simulink model "CM620C_MotAg0Meas"  (R2013b)
settings: Solver=FixedStepDiscrete  SolverMode=SingleTasking  StartTime=0.0  StopTime=1  FixedStep=0.0000625  RelTol=1e-3
values from neighbouring files (symbols this model uses):
  ARCHGLBPRM_2PI_ULS_F32 = DataDict.Constant    [CM620C_MotAg0Meas_DataDict.m]
  COEFFTBLELMSIZE_CNT_U08 = DataDict.Constant    [CM620C_MotAg0Meas_DataDict.m]
  COEFFTBLSIZE_CNT_U08 = DataDict.Constant    [CM620C_MotAg0Meas_DataDict.m]
  CORRNTBLAGSTEPSIZE_MATRAD_F32 = DataDict.Constant    [CM620C_MotAg0Meas_DataDict.m]
  CORRNTBLSIDXOFFS_CNT_U16 = DataDict.Constant    [CM620C_MotAg0Meas_DataDict.m]
  CORRNTBLSIZE_CNT_U16 = DataDict.Constant    [CM620C_MotAg0Meas_DataDict.m]
  CORRNTBLSIZEMASK_CNT_U08 = DataDict.Constant    [CM620C_MotAg0Meas_DataDict.m]
  MOTAG0ERRTHD_MOTREV_U0P16 = DataDict.Constant    [CM620C_MotAg0Meas_DataDict.m]
  MotAg0PrtclFlt = DataDict.NTC    [CM620C_MotAg0Meas_DataDict.m]
  MOTAG0PRTCLFLTFAILSTEP_CNT_U16 = DataDict.Constant    [CM620C_MotAg0Meas_DataDict.m]
  MOTAG0PRTCLFLTPASSSTEP_CNT_U16 = DataDict.Constant    [CM620C_MotAg0Meas_DataDict.m]
  MOTAGCPTLIMFLTMASK_CNT_U32 = DataDict.Constant    [CM620C_MotAg0Meas_DataDict.m]
  MOTAGDELTAPERCORRNPT_CNT_U16 = DataDict.Constant    [CM620C_MotAg0Meas_DataDict.m]
  MOTAGFLTMASK_CNT_U32 = DataDict.Constant    [CM620C_MotAg0Meas_DataDict.m]
  MOTAGIDXMASK_CNT_U16 = DataDict.Constant    [CM620C_MotAg0Meas_DataDict.m]
  MOTAGLIMMASK_CNT_S32 = DataDict.Constant    [CM620C_MotAg0Meas_DataDict.m]
  MOTAGMGNLIMFLTMASK_CNT_U32 = DataDict.Constant    [CM620C_MotAg0Meas_DataDict.m]
  MOTAGMINWAITPERD_CNT_U32 = DataDict.Constant    [CM620C_MotAg0Meas_DataDict.m]
  MOTAGOFFS_CNT_S32 = DataDict.Constant    [CM620C_MotAg0Meas_DataDict.m]
  MOTAGOVFFLTMASK_CNT_U32 = DataDict.Constant    [CM620C_MotAg0Meas_DataDict.m]
  MOTAGSPITRSMMASK_CNT_U32 = DataDict.Constant    [CM620C_MotAg0Meas_DataDict.m]
  MOTAGVLTGFLTMASK_CNT_U32 = DataDict.Constant    [CM620C_MotAg0Meas_DataDict.m]
  NOMOTAGFLTMASK_CNT_U32 = DataDict.Constant    [CM620C_MotAg0Meas_DataDict.m]
  READBUFADR_CNT_U32 = DataDict.Constant    [CM620C_MotAg0Meas_DataDict.m]
  READBUFIDX_CNT_U08 = DataDict.Constant    [CM620C_MotAg0Meas_DataDict.m]
  SNSRAGMASK_CNT_U32 = DataDict.Constant    [CM620C_MotAg0Meas_DataDict.m]
  SNSRCNTMASK_CNT_U32 = DataDict.Constant    [CM620C_MotAg0Meas_DataDict.m]
  SPIAGCNTREGIDX_CNT_U08 = DataDict.Constant    [CM620C_MotAg0Meas_DataDict.m]
  SPIAGREGIDX_CNT_U08 = DataDict.Constant    [CM620C_MotAg0Meas_DataDict.m]
  SPISTATREGIDX_CNT_U08 = DataDict.Constant    [CM620C_MotAg0Meas_DataDict.m]
  SPITURNCNTRREGIDX_CNT_U08 = DataDict.Constant    [CM620C_MotAg0Meas_DataDict.m]
  STRTPTRINITVAL_CNT_U32 = DataDict.Constant    [CM620C_MotAg0Meas_DataDict.m]
  STRTPTRPERVAL_CNT_U32 = DataDict.Constant    [CM620C_MotAg0Meas_DataDict.m]
  TURNCNTRHALFOFFS_CNT_S16 = DataDict.Constant    [CM620C_MotAg0Meas_DataDict.m]
  TURNCNTROFFS_CNT_S16 = DataDict.Constant    [CM620C_MotAg0Meas_DataDict.m]
  TURNCNTRREGMASK_CNT_U32 = DataDict.Constant    [CM620C_MotAg0Meas_DataDict.m]
  VLDMOTAGFLTMASK_CNT_U32 = DataDict.Constant    [CM620C_MotAg0Meas_DataDict.m]
undefined symbols (not defined in the file or in its folder): NtcSts1, sigbuilder_block
libraries: simulink x41, FloatToFixd x1, NxtrMax x1
(part 4 of 7)

== system CM620C_MotAg0Meas/MotAg0Meas/MotAg0MeasPer2/MotAg0Calcn/MotAg0Processing/Offset Compensation /Rt Offs Calcn ==
  MotAg3Mecl : Inport  RequirementInfo={} %GIDa_68f0f226_5b53_4cfc_a377_050a14e64919
  MotAg0SpiMecl : Inport  RequirementInfo={} %GIDa_5deca769_324c_4965_b2f5_c5a430060931  Port=2
  Action Port : ActionPort  ActionType=else
  CopyRight2 : Subsystem  Description=|  mask(Copyright Information){none=on}
      | Copyright info block.                                               
      |                                                                     
      | Place copyright information at the top of every subsystem in design.
      mask prompts: none "No parameters"
      mask help: Place copyright information at the top of every subsystem in design.
      mask Display:
      | NxtrConf = 'Nexteer Confidential';
      | 
      | sys = bdroot; %handle for the current model ("system")
      | first = get_param(sys,'Created');
      | first = first(end-3:end);  %year is last four digits
      | 
      | last = get_param(sys,'LastModifiedDate');
      | if isempty(last)
      |     last = datestr(now,'yyyy');
      | else
      |     last = last(end-3:end);
      | end
      | 
      | if strcmp(first,last)
      |     fprintf('%s -- Copyright %s Nexteer',NxtrConf,first)
      | else
      |     fprintf('%s -- %s%s- %s Nexteer',NxtrConf,char(169),first,last)
      | end
  Data Store Read1 : DataStoreRead  DataStoreName=MotAg0PrevOffs
  Data Type Conversion : DataTypeConversion  OutDataTypeStr=int32
  Data Type Conversion1 : DataTypeConversion  OutDataTypeStr=int32
  Subtract : Sum  Inputs=+-
  MotAg0Offs : Outport
  MotAg0RtOffs : Outport  Port=2
  wires:
  MotAg3Mecl/1 -> Data Type Conversion/1
  Subtract/1 -> MotAg0RtOffs/1
  Data Type Conversion1/1 -> Subtract/2
  Data Type Conversion/1 -> Subtract/1
  MotAg0SpiMecl/1 -> Data Type Conversion1/1
  Data Store Read1/1 -> MotAg0Offs/1

== system CM620C_MotAg0Meas/MotAg0Meas/MotAg0MeasPer2/MotAg0Calcn/MotAg0Processing/SPI  Motor Angle Calcn/CopyRight1 ==

== system CM620C_MotAg0Meas/MotAg0Meas/MotAg0MeasPer2/MotAg0Calcn/MotAg0Processing/SPI  Motor Angle Calcn/Polarity Correction ==
  MotAg0RawSpiMecl : Inport
  MotAgMecl0Polarity : Inport  Port=2
  CopyRight1 : Subsystem  Description=|  mask(Copyright Information){none=on}
      | Copyright info block.                                               
      |                                                                     
      | Place copyright information at the top of every subsystem in design.
      mask prompts: none "No parameters"
      mask help: Place copyright information at the top of every subsystem in design.
      mask Display:
      | NxtrConf = 'Nexteer Confidential';
      | 
      | sys = bdroot; %handle for the current model ("system")
      | first = get_param(sys,'Created');
      | first = first(end-3:end);  %year is last four digits
      | 
      | last = get_param(sys,'LastModifiedDate');
      | if isempty(last)
      |     last = datestr(now,'yyyy');
      | else
      |     last = last(end-3:end);
      | end
      | 
      | if strcmp(first,last)
      |     fprintf('%s -- Copyright %s Nexteer',NxtrConf,first)
      | else
      |     fprintf('%s -- %s%s- %s Nexteer',NxtrConf,char(169),first,last)
      | end
  Data Store Write : DataStoreWrite  DataStoreName=dMotAg0MeasMotAg0SpiMecl
  If : If  IfExpression=u1 < 0
  Merge : Merge
  Negative Polarity : Subsystem  TreatAsAtomicUnit=on
  Positive Polarity : Subsystem  TreatAsAtomicUnit=on
  MotAg0SpiMecl : Outport
  wires:
  MotAgMecl0Polarity/1 -> If/1
  MotAg0RawSpiMecl/1 -> Negative Polarity/1(MotAg0RawSpiMecl), Positive Polarity/1(MotAg0RawSpiMecl)
  If/1 -> Negative Polarity/Action
  If/2 -> Positive Polarity/Action
  Negative Polarity/1(MotAg0SpiPolarityCorrd) -> Merge/1
  Positive Polarity/1(MotAg0SpiPolarityCorrd) -> Merge/2
  Merge/1 -> MotAg0SpiMecl/1, Data Store Write/1

== system CM620C_MotAg0Meas/MotAg0Meas/MotAg0MeasPer2/MotAg0Calcn/MotAg0Processing/SPI IIF Motor Angle/CopyRight2 ==

== system CM620C_MotAg0Meas/MotAg0Meas/MotAg0MeasPer2/MotAg0Calcn/MotAg0Processing/SPI IIF Motor Angle/SpiMotAgCnt ==
  note: Square Pulse per angle step. 14 bit- 16384 steps per full roation
  MotAg0AgCntReg : Inport
  14-bit Count Value : simulink/Logic and Bit Operations/Bitwise Operator  logicop=AND  UseBitMask=off  NumInputPorts=2  BitMask=SNSRVLTGFLTMASK_CNT_U32  BitMaskRealWorld=Stored Integer
  16383 : Constant  Value=SNSRCNTMASK_CNT_U32
  CopyRight2 : Subsystem  Description=|  mask(Copyright Information){none=on}
      | Copyright info block.                                               
      |                                                                     
      | Place copyright information at the top of every subsystem in design.
      mask prompts: none "No parameters"
      mask help: Place copyright information at the top of every subsystem in design.
      mask Display:
      | NxtrConf = 'Nexteer Confidential';
      | 
      | sys = bdroot; %handle for the current model ("system")
      | first = get_param(sys,'Created');
      | first = first(end-3:end);  %year is last four digits
      | 
      | last = get_param(sys,'LastModifiedDate');
      | if isempty(last)
      |     last = datestr(now,'yyyy');
      | else
      |     last = last(end-3:end);
      | end
      | 
      | if strcmp(first,last)
      |     fprintf('%s -- Copyright %s Nexteer',NxtrConf,first)
      | else
      |     fprintf('%s -- %s%s- %s Nexteer',NxtrConf,char(169),first,last)
      | end
  Data Type Conversion : DataTypeConversion  OutDataTypeStr=uint16
  Left Shift 2 Bits - p16 : ArithShift  BitShiftNumber=2  BitShiftDirection=Left
  Scope : Scope  NumInputPorts=2
      settings: YMin=0~0  YMax=17000~70000  SaveName=ScopeData4
  MotAg0SpiCntr : Outport
  wires:
  MotAg0AgCntReg/1 -> 14-bit Count Value/1
  16383/1 -> 14-bit Count Value/2
  14-bit Count Value/1 -> Data Type Conversion/1
  Left Shift 2 Bits - p16/1 -> MotAg0SpiCntr/1, Scope/2
  Data Type Conversion/1 -> Left Shift 2 Bits - p16/1, Scope/1

== system CM620C_MotAg0Meas/MotAg0Meas/MotAg0MeasPer2/MotAg0Calcn/MotAg0Processing/Turns Counter Calcn/CopyRight2 ==

== system CM620C_MotAg0Meas/MotAg0Meas/MotAg0MeasPer2/MotAg0Calcn/MotAg0Processing/Turns Counter Calcn/Negative Number ==
  Action Port : ActionPort  ActionType=then
  512 : Constant  Value=TURNCNTROFFS_CNT_S16
  CopyRight2 : Subsystem  Description=|  mask(Copyright Information){none=on}
      | Copyright info block.                                               
      |                                                                     
      | Place copyright information at the top of every subsystem in design.
      mask prompts: none "No parameters"
      mask help: Place copyright information at the top of every subsystem in design.
      mask Display:
      | NxtrConf = 'Nexteer Confidential';
      | 
      | sys = bdroot; %handle for the current model ("system")
      | first = get_param(sys,'Created');
      | first = first(end-3:end);  %year is last four digits
      | 
      | last = get_param(sys,'LastModifiedDate');
      | if isempty(last)
      |     last = datestr(now,'yyyy');
      | else
      |     last = last(end-3:end);
      | end
      | 
      | if strcmp(first,last)
      |     fprintf('%s -- Copyright %s Nexteer',NxtrConf,first)
      | else
      |     fprintf('%s -- %s%s- %s Nexteer',NxtrConf,char(169),first,last)
      | end
  Out1 : Outport
  wires:
  512/1 -> Out1/1

== system CM620C_MotAg0Meas/MotAg0Meas/MotAg0MeasPer2/MotAg0Calcn/MotAg0Processing/Turns Counter Calcn/Positive Number ==
  Action Port : ActionPort  ActionType=else
  Constant3 : Constant  Value=0  OutDataTypeStr=int16
  CopyRight2 : Subsystem  Description=|  mask(Copyright Information){none=on}
      | Copyright info block.                                               
      |                                                                     
      | Place copyright information at the top of every subsystem in design.
      mask prompts: none "No parameters"
      mask help: Place copyright information at the top of every subsystem in design.
      mask Display:
      | NxtrConf = 'Nexteer Confidential';
      | 
      | sys = bdroot; %handle for the current model ("system")
      | first = get_param(sys,'Created');
      | first = first(end-3:end);  %year is last four digits
      | 
      | last = get_param(sys,'LastModifiedDate');
      | if isempty(last)
      |     last = datestr(now,'yyyy');
      | else
      |     last = last(end-3:end);
      | end
      | 
      | if strcmp(first,last)
      |     fprintf('%s -- Copyright %s Nexteer',NxtrConf,first)
      | else
      |     fprintf('%s -- %s%s- %s Nexteer',NxtrConf,char(169),first,last)
      | end
  Out1 : Outport
  wires:
  Constant3/1 -> Out1/1

== system CM620C_MotAg0Meas/MotAg0Meas/MotAg0MeasPer2/MotAg0Calcn/SpiRx/Data/CopyRight2 ==

== system CM620C_MotAg0Meas/MotAg0Meas/MotAg0MeasPer3/Initial Check/IdleState SendTx/Flt Cntr Ena/CopyRight2 ==

== system CM620C_MotAg0Meas/MotAg0Meas/MotAg0MeasPer3/Initial Check/IdleState SendTx/Flt Cntr Ena/Wrap back to 0 ==
  Action Port : ActionPort  ActionType=then
  Constant : Constant  Value=0  OutDataTypeStr=uint16
  CopyRight2 : Subsystem  Description=|  mask(Copyright Information){none=on}
      | Copyright info block.                                               
      |                                                                     
      | Place copyright information at the top of every subsystem in design.
      mask prompts: none "No parameters"
      mask help: Place copyright information at the top of every subsystem in design.
      mask Display:
      | NxtrConf = 'Nexteer Confidential';
      | 
      | sys = bdroot; %handle for the current model ("system")
      | first = get_param(sys,'Created');
      | first = first(end-3:end);  %year is last four digits
      | 
      | last = get_param(sys,'LastModifiedDate');
      | if isempty(last)
      |     last = datestr(now,'yyyy');
      | else
      |     last = last(end-3:end);
      | end
      | 
      | if strcmp(first,last)
      |     fprintf('%s -- Copyright %s Nexteer',NxtrConf,first)
      | else
      |     fprintf('%s -- %s%s- %s Nexteer',NxtrConf,char(169),first,last)
      | end
  FltCntr_u16 : Outport
  wires:
  Constant/1 -> FltCntr_u16/1

== system CM620C_MotAg0Meas/MotAg0Meas/MotAg0MeasPer3/Initial Check/IdleState SendTx/Flt Cntr Ena/i++ ==
  Action Port : ActionPort  ActionType=else
  Add : Sum
  Constant : Constant  OutDataTypeStr=uint16
  CopyRight2 : Subsystem  Description=|  mask(Copyright Information){none=on}
      | Copyright info block.                                               
      |                                                                     
      | Place copyright information at the top of every subsystem in design.
      mask prompts: none "No parameters"
      mask help: Place copyright information at the top of every subsystem in design.
      mask Display:
      | NxtrConf = 'Nexteer Confidential';
      | 
      | sys = bdroot; %handle for the current model ("system")
      | first = get_param(sys,'Created');
      | first = first(end-3:end);  %year is last four digits
      | 
      | last = get_param(sys,'LastModifiedDate');
      | if isempty(last)
      |     last = datestr(now,'yyyy');
      | else
      |     last = last(end-3:end);
      | end
      | 
      | if strcmp(first,last)
      |     fprintf('%s -- Copyright %s Nexteer',NxtrConf,first)
      | else
      |     fprintf('%s -- %s%s- %s Nexteer',NxtrConf,char(169),first,last)
      | end
  Data Store Read : DataStoreRead  DataStoreName=MotAg0PrevSpiErrFltCntr
  FltCntr_u16 : Outport
  wires:
  Constant/1 -> Add/1
  Data Store Read/1 -> Add/2
  Add/1 -> FltCntr_u16/1

== system CM620C_MotAg0Meas/MotAg0Meas/MotAg0MeasPer3/Initial Check/IdleState SendTx/MotAg0Sync/CopyRight2 ==

== system CM620C_MotAg0Meas/MotAg0Meas/MotAg0MeasPer3/Initial Check/IdleState SendTx/MotAg0Sync/GetMotAg3Mecl ==
  CopyRight2 : Subsystem  Description=|  mask(Copyright Information){none=on}
      | Copyright info block.                                               
      |                                                                     
      | Place copyright information at the top of every subsystem in design.
      mask prompts: none "No parameters"
      mask help: Place copyright information at the top of every subsystem in design.
      mask Display:
      | NxtrConf = 'Nexteer Confidential';
      | 
      | sys = bdroot; %handle for the current model ("system")
      | first = get_param(sys,'Created');
      | first = first(end-3:end);  %year is last four digits
      | 
      | last = get_param(sys,'LastModifiedDate');
      | if isempty(last)
      |     last = datestr(now,'yyyy');
      | else
      |     last = last(end-3:end);
      | end
      | 
      | if strcmp(first,last)
      |     fprintf('%s -- Copyright %s Nexteer',NxtrConf,first)
      | else
      |     fprintf('%s -- %s%s- %s Nexteer',NxtrConf,char(169),first,last)
      | end
  SimulationOnly : DataStoreRead  DataStoreName=SimulatedIIFAg
  MotAg3Mecl : Outport
  wires:
  SimulationOnly/1 -> MotAg3Mecl/1

== system CM620C_MotAg0Meas/MotAg0Meas/MotAg0MeasPer3/Initial Check/IdleState SendTx/MotAg0Sync/IoHwAb_SetFctGpioMotAg0 ==
  CopyRight2 : Subsystem  Description=|  mask(Copyright Information){none=on}
      | Copyright info block.                                               
      |                                                                     
      | Place copyright information at the top of every subsystem in design.
      mask prompts: none "No parameters"
      mask help: Place copyright information at the top of every subsystem in design.
      mask Display:
      | NxtrConf = 'Nexteer Confidential';
      | 
      | sys = bdroot; %handle for the current model ("system")
      | first = get_param(sys,'Created');
      | first = first(end-3:end);  %year is last four digits
      | 
      | last = get_param(sys,'LastModifiedDate');
      | if isempty(last)
      |     last = datestr(now,'yyyy');
      | else
      |     last = last(end-3:end);
      | end
      | 
      | if strcmp(first,last)
      |     fprintf('%s -- Copyright %s Nexteer',NxtrConf,first)
      | else
      |     fprintf('%s -- %s%s- %s Nexteer',NxtrConf,char(169),first,last)
      | end

== system CM620C_MotAg0Meas/MotAg0Meas/MotAg0MeasPer3/Initial Check/IdleState SendTx/MotAg0Sync/IoHwAb_SetFctPrphlMotAg0 ==
  CopyRight2 : Subsystem  Description=|  mask(Copyright Information){none=on}
      | Copyright info block.                                               
      |                                                                     
      | Place copyright information at the top of every subsystem in design.
      mask prompts: none "No parameters"
      mask help: Place copyright information at the top of every subsystem in design.
      mask Display:
      | NxtrConf = 'Nexteer Confidential';
      | 
      | sys = bdroot; %handle for the current model ("system")
      | first = get_param(sys,'Created');
      | first = first(end-3:end);  %year is last four digits
      | 
      | last = get_param(sys,'LastModifiedDate');
      | if isempty(last)
      |     last = datestr(now,'yyyy');
      | else
      |     last = last(end-3:end);
      | end
      | 
      | if strcmp(first,last)
      |     fprintf('%s -- Copyright %s Nexteer',NxtrConf,first)
      | else
      |     fprintf('%s -- %s%s- %s Nexteer',NxtrConf,char(169),first,last)
      | end

== system CM620C_MotAg0Meas/MotAg0Meas/MotAg0MeasPer3/Initial Check/IdleState SendTx/MotAg0Sync/Set Chip Select High ==
  "  " : Constant  OutDataTypeStr=boolean
  CopyRight2 : Subsystem  Description=|  mask(Copyright Information){none=on}
      | Copyright info block.                                               
      |                                                                     
      | Place copyright information at the top of every subsystem in design.
      mask prompts: none "No parameters"
      mask help: Place copyright information at the top of every subsystem in design.
      mask Display:
      | NxtrConf = 'Nexteer Confidential';
      | 
      | sys = bdroot; %handle for the current model ("system")
      | first = get_param(sys,'Created');
      | first = first(end-3:end);  %year is last four digits
      | 
      | last = get_param(sys,'LastModifiedDate');
      | if isempty(last)
      |     last = datestr(now,'yyyy');
      | else
      |     last = last(end-3:end);
      | end
      | 
      | if strcmp(first,last)
      |     fprintf('%s -- Copyright %s Nexteer',NxtrConf,first)
      | else
      |     fprintf('%s -- %s%s- %s Nexteer',NxtrConf,char(169),first,last)
      | end
  IoHwAb_SetGpioMotAg0Cs : Subsystem  TreatAsAtomicUnit=on
  wires:
  "  "/1 -> IoHwAb_SetGpioMotAg0Cs/1(PinSt)

== system CM620C_MotAg0Meas/MotAg0Meas/MotAg0MeasPer3/Initial Check/IdleState SendTx/MotAg0Sync/Set Chip Select Low ==
  "  " : Constant  Value=0  OutDataTypeStr=boolean
  CopyRight2 : Subsystem  Description=|  mask(Copyright Information){none=on}
      | Copyright info block.                                               
      |                                                                     
      | Place copyright information at the top of every subsystem in design.
      mask prompts: none "No parameters"
      mask help: Place copyright information at the top of every subsystem in design.
      mask Display:
      | NxtrConf = 'Nexteer Confidential';
      | 
      | sys = bdroot; %handle for the current model ("system")
      | first = get_param(sys,'Created');
      | first = first(end-3:end);  %year is last four digits
      | 
      | last = get_param(sys,'LastModifiedDate');
      | if isempty(last)
      |     last = datestr(now,'yyyy');
      | else
      |     last = last(end-3:end);
      | end
      | 
      | if strcmp(first,last)
      |     fprintf('%s -- Copyright %s Nexteer',NxtrConf,first)
      | else
      |     fprintf('%s -- %s%s- %s Nexteer',NxtrConf,char(169),first,last)
      | end
  IoHwAb_SetGpioMotAg0Cs : Subsystem  TreatAsAtomicUnit=on
  wires:
  "  "/1 -> IoHwAb_SetGpioMotAg0Cs/1(PinSt)

== system CM620C_MotAg0Meas/MotAg0Meas/MotAg0MeasPer3/Initial Check/IdleState SendTx/MotAg0Sync/SpiTx ==
  note: Send Tx Data in the following order. Start Pointer - Number of messeges.
  note: CSIH1SOP - 0:6 bits (Start Pointer)
      | 0001000 = 8
      | CSIH1ND 16:23 bits (No. Of Data)
      | 00001011 = 12
      | CSIH1BTST - 31st bit (Issue Transfer)
      | 1
      | Dec = 2148270088
  CopyRight2 : Subsystem  Description=|  mask(Copyright Information){none=on}
      | Copyright info block.                                               
      |                                                                     
      | Place copyright information at the top of every subsystem in design.
      mask prompts: none "No parameters"
      mask help: Place copyright information at the top of every subsystem in design.
      mask Display:
      | NxtrConf = 'Nexteer Confidential';
      | 
      | sys = bdroot; %handle for the current model ("system")
      | first = get_param(sys,'Created');
      | first = first(end-3:end);  %year is last four digits
      | 
      | last = get_param(sys,'LastModifiedDate');
      | if isempty(last)
      |     last = datestr(now,'yyyy');
      | else
      |     last = last(end-3:end);
      | end
      | 
      | if strcmp(first,last)
      |     fprintf('%s -- Copyright %s Nexteer',NxtrConf,first)
      | else
      |     fprintf('%s -- %s%s- %s Nexteer',NxtrConf,char(169),first,last)
      | end
  RegOutpCSIH1MCTL2 : Terminator
  Start Pointer No. of Data : Constant  Value=STRTPTRPERVAL_CNT_U32
  wires:
  Start Pointer No. of Data/1 -> RegOutpCSIH1MCTL2/1

== system CM620C_MotAg0Meas/MotAg0Meas/MotAg0MeasPer3/Initial Check/IdleState SendTx/MotAg0Sync/Wait for 2us ==
  note: 1 count = 1us
      | 2 Counts = 2us (Min Wait Per)
  note: Call Once
  note: Run untill output of this is >= Minimum of 2us (Constant Defined as 2 counts = 2 us)
  2 Counts : Constant  Value=MOTAGMINWAITPERD_CNT_U32
  CopyRight2 : Subsystem  Description=|  mask(Copyright Information){none=on}
      | Copyright info block.                                               
      |                                                                     
      | Place copyright information at the top of every subsystem in design.
      mask prompts: none "No parameters"
      mask help: Place copyright information at the top of every subsystem in design.
      mask Display:
      | NxtrConf = 'Nexteer Confidential';
      | 
      | sys = bdroot; %handle for the current model ("system")
      | first = get_param(sys,'Created');
      | first = first(end-3:end);  %year is last four digits
      | 
      | last = get_param(sys,'LastModifiedDate');
      | if isempty(last)
      |     last = datestr(now,'yyyy');
      | else
      |     last = last(end-3:end);
      | end
      | 
      | if strcmp(first,last)
      |     fprintf('%s -- Copyright %s Nexteer',NxtrConf,first)
      | else
      |     fprintf('%s -- %s%s- %s Nexteer',NxtrConf,char(169),first,last)
      | end
  GetRefTmr1MicroSec32bit : Subsystem  TreatAsAtomicUnit=on
  GetTiSpan1MicroSec32bit : Subsystem
  Terminator1 : Terminator
  Terminator2 : Terminator
  wires:
  GetRefTmr1MicroSec32bit/1(RefTmr) -> GetTiSpan1MicroSec32bit/1(RefTmr)
  GetTiSpan1MicroSec32bit/1(TiSpan) -> Terminator1/1
  2 Counts/1 -> Terminator2/1

== system CM620C_MotAg0Meas/MotAg0Meas/MotAg0MeasPer3/Initial Check/InitTxCommunication going on Wait/Last Flt Cntr /CopyRight2 ==

== system CM620C_MotAg0Meas/MotAg0Meas/MotAg0MeasInit1/Compute Correction Table/NVM Ok/Calculate Correction Table/Build Wave/CopyRight2 ==

== system CM620C_MotAg0Meas/MotAg0Meas/MotAg0MeasInit1/Compute Correction Table/NVM Ok/Calculate Correction Table/Build Wave/Reconstructed Waveform Processing ==
  N : Inport
  Assignment : Assignment  IndexMode=Zero-based  IndexOptions=Index vector (port)  Indices=1  OutputSizes=1
  Constant : Constant  Value=COEFFTBLSIZE_CNT_U08
  Constant1 : Constant  Value=CORRNTBLAGSTEPSIZE_MATRAD_F32
  CopyRight2 : Subsystem  Description=|  mask(Copyright Information){none=on}
      | Copyright info block.                                               
      |                                                                     
      | Place copyright information at the top of every subsystem in design.
      mask prompts: none "No parameters"
      mask help: Place copyright information at the top of every subsystem in design.
      mask Display:
      | NxtrConf = 'Nexteer Confidential';
      | 
      | sys = bdroot; %handle for the current model ("system")
      | first = get_param(sys,'Created');
      | first = first(end-3:end);  %year is last four digits
      | 
      | last = get_param(sys,'LastModifiedDate');
      | if isempty(last)
      |     last = datestr(now,'yyyy');
      | else
      |     last = last(end-3:end);
      | end
      | 
      | if strcmp(first,last)
      |     fprintf('%s -- Copyright %s Nexteer',NxtrConf,first)
      | else
      |     fprintf('%s -- %s%s- %s Nexteer',NxtrConf,char(169),first,last)
      | end
  Data Store Read : DataStoreRead  DataStoreName=ReconstructedWaveform_RevM_f32
  Data Store Write : DataStoreWrite  DataStoreName=ReconstructedWaveform_RevM_f32
  Data Type Conversion : DataTypeConversion  OutDataTypeStr=single
  Data Type Conversion1 : DataTypeConversion  OutDataTypeStr=int8
  For Iterator : ForIterator  ResetStates=reset  IterationSource=external  IndexMode=Zero-based  IterationVariableDataType=int16
  Harmonic Coefficient Processing : Subsystem  TreatAsAtomicUnit=on
  Product : Product
  Subtract 1 because the first order is not included : Bias  Bias=-1
  wires:
  Constant/1 -> Data Type Conversion1/1
  N/1 -> For Iterator/1
  For Iterator/1 -> Data Type Conversion/1, Assignment/3
  Data Type Conversion/1 -> Product/1
  Constant1/1 -> Product/2
  Product/1 -> Harmonic Coefficient Processing/1(HarmAngle)
  Data Store Read/1 -> Assignment/1
  Subtract 1 because the first order is not included/1 -> Harmonic Coefficient Processing/2(Coefficient Table Size)
  Data Type Conversion1/1 -> Subtract 1 because the first order is not included/1
  Harmonic Coefficient Processing/1(Reconstructed Waveform Element) -> Assignment/2
  Assignment/1 -> Data Store Write/1

== system CM620C_MotAg0Meas/MotAg0Meas/MotAg0MeasInit1/Compute Correction Table/NVM Ok/Calculate Correction Table/Change Correction Coordinate/CopyRight2 ==

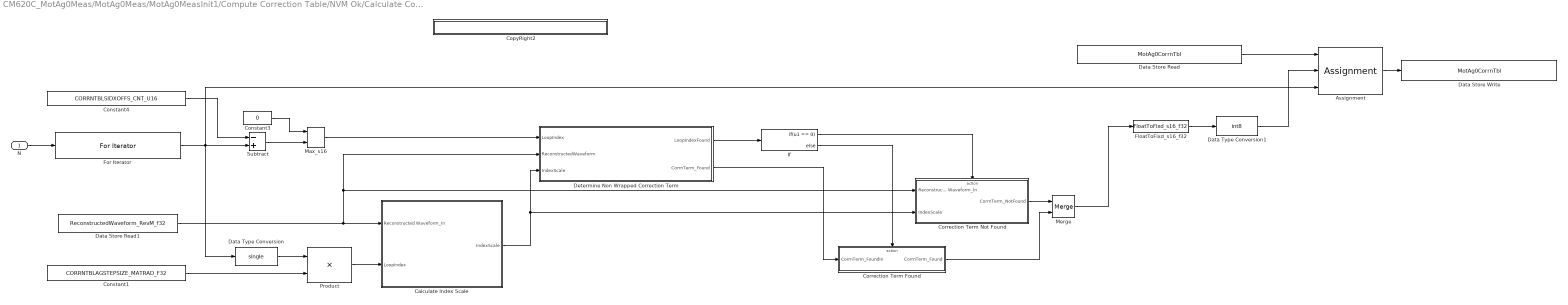
== system CM620C_MotAg0Meas/MotAg0Meas/MotAg0MeasInit1/Compute Correction Table/NVM Ok/Calculate Correction Table/Change Correction Coordinate/Waveform Coordinate Change ==
  N : Inport
  Assignment : Assignment  IndexMode=Zero-based  IndexOptions=Index vector (port)  Indices=1  OutputSizes=1
  Calculate Index Scale : Subsystem  TreatAsAtomicUnit=on
  Constant1 : Constant  Value=CORRNTBLAGSTEPSIZE_MATRAD_F32
  Constant3 : Constant  Value=0  OutDataTypeStr=int16
  Constant4 : Constant  Value=CORRNTBLSIDXOFFS_CNT_U16
  CopyRight2 : Subsystem  Description=|  mask(Copyright Information){none=on}
      | Copyright info block.                                               
      |                                                                     
      | Place copyright information at the top of every subsystem in design.
      mask prompts: none "No parameters"
      mask help: Place copyright information at the top of every subsystem in design.
      mask Display:
      | NxtrConf = 'Nexteer Confidential';
      | 
      | sys = bdroot; %handle for the current model ("system")
      | first = get_param(sys,'Created');
      | first = first(end-3:end);  %year is last four digits
      | 
      | last = get_param(sys,'LastModifiedDate');
      | if isempty(last)
      |     last = datestr(now,'yyyy');
      | else
      |     last = last(end-3:end);
      | end
      | 
      | if strcmp(first,last)
      |     fprintf('%s -- Copyright %s Nexteer',NxtrConf,first)
      | else
      |     fprintf('%s -- %s%s- %s Nexteer',NxtrConf,char(169),first,last)
      | end
  Correction Term Found : Subsystem  TreatAsAtomicUnit=on
  Correction Term Not Found : Subsystem  TreatAsAtomicUnit=on
  Data Store Read : DataStoreRead  DataStoreName=MotAg0CorrnTbl
  Data Store Read1 : DataStoreRead  DataStoreName=ReconstructedWaveform_RevM_f32
  Data Store Write : DataStoreWrite  DataStoreName=MotAg0CorrnTbl
  Data Type Conversion : DataTypeConversion  OutDataTypeStr=single
  Data Type Conversion1 : DataTypeConversion  OutDataTypeStr=int8
  Determine Non Wrapped Correction Term : Subsystem  TreatAsAtomicUnit=on
  FloatToFixd_s16_f32 : FloatToFixd/FloatToFixd_s16_f32  Param1=12
  For Iterator : ForIterator  ResetStates=reset  IterationSource=external  IndexMode=Zero-based  IterationVariableDataType=int16
  If : If  IfExpression=u1 == 0
  Max_s16 : NxtrMax/Max_s16  SFunctionSpec="int16 y1 = Max_s16( int16 u1,  int16 u2)"
      settings: AttributesFormatString=%<Name>
  Merge : Merge
  Product : Product
  Subtract : Sum  Inputs=-+  OutDataTypeStr=int16
  wires:
  Constant1/1 -> Product/2
  Data Type Conversion/1 -> Product/1
  For Iterator/1 -> Data Type Conversion/1, Assignment/3, Subtract/2
  N/1 -> For Iterator/1
  Data Store Read1/1 -> Correction Term Not Found/1(Reconstructed Waveform_In), Determine Non Wrapped Correction Term/2(ReconstructedWaveform), Calculate Index Scale/1(Reconstructed Waveform_In)
  Product/1 -> Calculate Index Scale/2(LoopIndex)
  Calculate Index Scale/1(IndexScale) -> Correction Term Not Found/2(IndexScale), Determine Non Wrapped Correction Term/3(IndexScale)
  Constant3/1 -> Max_s16/1
  Subtract/1 -> Max_s16/2
  Constant4/1 -> Subtract/1
  Max_s16/1 -> Determine Non Wrapped Correction Term/1(LoopIndex)
  Determine Non Wrapped Correction Term/1(LoopIndexFound) -> If/1
  If/1 -> Correction Term Not Found/Action
  If/2 -> Correction Term Found/Action
  Determine Non Wrapped Correction Term/2(CorrnTerm_Found) -> Correction Term Found/1(CorrnTerm_FoundIn)
  Data Store Read/1 -> Assignment/1
  Correction Term Not Found/1(CorrnTerm_NotFound) -> Merge/1
  Correction Term Found/1(CorrnTerm_Found) -> Merge/2
  Merge/1 -> FloatToFixd_s16_f32/1
  Assignment/1 -> Data Store Write/1
  FloatToFixd_s16_f32/1 -> Data Type Conversion1/1
  Data Type Conversion1/1 -> Assignment/2

== system CM620C_MotAg0Meas/MotAg0Meas/MotAg0MeasPer2/MotAg0Calcn/MotAg0Processing/Diagnostics/ Qualifier Sts/CopyRight2 ==

== system CM620C_MotAg0Meas/MotAg0Meas/MotAg0MeasPer2/MotAg0Calcn/MotAg0Processing/Diagnostics/ Qualifier Sts/GetNtcQlfr ==
  NtcNr : Inport
  CopyRight2 : Subsystem  Description=|  mask(Copyright Information){none=on}
      | Copyright info block.                                               
      |                                                                     
      | Place copyright information at the top of every subsystem in design.
      mask prompts: none "No parameters"
      mask help: Place copyright information at the top of every subsystem in design.
      mask Display:
      | NxtrConf = 'Nexteer Confidential';
      | 
      | sys = bdroot; %handle for the current model ("system")
      | first = get_param(sys,'Created');
      | first = first(end-3:end);  %year is last four digits
      | 
      | last = get_param(sys,'LastModifiedDate');
      | if isempty(last)
      |     last = datestr(now,'yyyy');
      | else
      |     last = last(end-3:end);
      | end
      | 
      | if strcmp(first,last)
      |     fprintf('%s -- Copyright %s Nexteer',NxtrConf,first)
      | else
      |     fprintf('%s -- %s%s- %s Nexteer',NxtrConf,char(169),first,last)
      | end
  Data Store Read : DataStoreRead  DataStoreName=NtcQlfr
  Terminator : Terminator
  NtcQlfr : Outport
  wires:
  NtcNr/1 -> Terminator/1
  Data Store Read/1 -> NtcQlfr/1

== system CM620C_MotAg0Meas/MotAg0Meas/MotAg0MeasPer2/MotAg0Calcn/MotAg0Processing/Diagnostics/ Qualifier Sts/NtcSts and DebStep Calcn ==
  NtcStInfo : Inport  OutDataTypeStr=uint8
  CopyRight2 : Subsystem  Description=|  mask(Copyright Information){none=on}
      | Copyright info block.                                               
      |                                                                     
      | Place copyright information at the top of every subsystem in design.
      mask prompts: none "No parameters"
      mask help: Place copyright information at the top of every subsystem in design.
      mask Display:
      | NxtrConf = 'Nexteer Confidential';
      | 
      | sys = bdroot; %handle for the current model ("system")
      | first = get_param(sys,'Created');
      | first = first(end-3:end);  %year is last four digits
      | 
      | last = get_param(sys,'LastModifiedDate');
      | if isempty(last)
      |     last = datestr(now,'yyyy');
      | else
      |     last = last(end-3:end);
      | end
      | 
      | if strcmp(first,last)
      |     fprintf('%s -- Copyright %s Nexteer',NxtrConf,first)
      | else
      |     fprintf('%s -- %s%s- %s Nexteer',NxtrConf,char(169),first,last)
      | end
  If : If
  Merge : Merge
  Merge1 : Merge
  N Step : Subsystem  RequirementInfo="{'linktype_rmi_doors' '00011b4e (/ESG Group/FDD Module Requirements/EA4 Specific/CM620C_MotAg0Meas)' '#CM620C_30' 'true' 'REQ:  CM620C_30' '' } %GIDa_c8512ee7_8c31_4537_a0b8_359b7e9dee0f"  TreatAsAtomicUnit=on
  P Step : Subsystem  TreatAsAtomicUnit=on
  NtcSts : Outport
  DebStep : Outport  Port=2  OutDataTypeStr=uint16
  wires:
  NtcStInfo/1 -> If/1
  If/1 -> P Step/Action
  If/2 -> N Step/Action
  Merge/1 -> DebStep/1
  P Step/1(NtcSts) -> Merge1/1
  N Step/1(NtcSts) -> Merge1/2
  P Step/2(DebStep) -> Merge/1
  N Step/2(DebStep) -> Merge/2
  Merge1/1 -> NtcSts/1

== system CM620C_MotAg0Meas/MotAg0Meas/MotAg0MeasPer2/MotAg0Calcn/MotAg0Processing/Diagnostics/ Qualifier Sts/SetNtcSts ==
  note: Only pass values 2 or 3 as input to NtcSts.
      | 2: PrePassd
      | 3: PreFaild
  NtcNr : Inport
  NtcStInfo : Inport  Port=2
  NtcSts : Inport  Port=3  OutDataTypeStr=Enum: NtcSts1
  DebStep : Inport  Port=4  OutDataTypeStr=uint16
  CopyRight2 : Subsystem  Description=|  mask(Copyright Information){none=on}
      | Copyright info block.                                               
      |                                                                     
      | Place copyright information at the top of every subsystem in design.
      mask prompts: none "No parameters"
      mask help: Place copyright information at the top of every subsystem in design.
      mask Display:
      | NxtrConf = 'Nexteer Confidential';
      | 
      | sys = bdroot; %handle for the current model ("system")
      | first = get_param(sys,'Created');
      | first = first(end-3:end);  %year is last four digits
      | 
      | last = get_param(sys,'LastModifiedDate');
      | if isempty(last)
      |     last = datestr(now,'yyyy');
      | else
      |     last = last(end-3:end);
      | end
      | 
      | if strcmp(first,last)
      |     fprintf('%s -- Copyright %s Nexteer',NxtrConf,first)
      | else
      |     fprintf('%s -- %s%s- %s Nexteer',NxtrConf,char(169),first,last)
      | end
  Data Store Write1 : DataStoreWrite  RequirementInfo={} %GIDa_134437e5_1119_46ed_80d5_e3e67bdcad62  DataStoreName=NtcQlfr
  Ground : Ground
  ISO Fault Debounce Design : Stateflow chart  TreatAsAtomicUnit=on
      settings: AttributesFormatString=|
      | Simulation Purpose Only.
      | Do Not Code this block
      | Diagnostic Manager Owns this requirement
  Only here because I could not get model to run with enumerations in the stateflow diagram : DataTypeConversion  OutDataTypeStr=uint8
  Terminator : Terminator
  Terminator1 : Terminator
  wires:
  NtcSts/1 -> Only here because I could not get model to run with enumerations in the stateflow diagram/1
  NtcNr/1 -> Terminator/1
  NtcStInfo/1 -> Terminator1/1
  Only here because I could not get model to run with enumerations in the stateflow diagram/1 -> ISO Fault Debounce Design/1(NtcSts)
  DebStep/1 -> ISO Fault Debounce Design/2(DebStep)
  ISO Fault Debounce Design/1(Qualifier) -> Data Store Write1/1
  Ground/1 -> ISO Fault Debounce Design/3(SvcClr)

== system CM620C_MotAg0Meas/MotAg0Meas/MotAg0MeasPer2/MotAg0Calcn/MotAg0Processing/Diagnostics/Rolling Counter/CopyRight2 ==

== system CM620C_MotAg0Meas/MotAg0Meas/MotAg0MeasPer2/MotAg0Calcn/MotAg0Processing/Diagnostics/Rolling Counter/Test Faild ==
  Action Port : ActionPort  ActionType=else
  CopyRight2 : Subsystem  Description=|  mask(Copyright Information){none=on}
      | Copyright info block.                                               
      |                                                                     
      | Place copyright information at the top of every subsystem in design.
      mask prompts: none "No parameters"
      mask help: Place copyright information at the top of every subsystem in design.
      mask Display:
      | NxtrConf = 'Nexteer Confidential';
      | 
      | sys = bdroot; %handle for the current model ("system")
      | first = get_param(sys,'Created');
      | first = first(end-3:end);  %year is last four digits
      | 
      | last = get_param(sys,'LastModifiedDate');
      | if isempty(last)
      |     last = datestr(now,'yyyy');
      | else
      |     last = last(end-3:end);
      | end
      | 
      | if strcmp(first,last)
      |     fprintf('%s -- Copyright %s Nexteer',NxtrConf,first)
      | else
      |     fprintf('%s -- %s%s- %s Nexteer',NxtrConf,char(169),first,last)
      | end
  Data Store Read : DataStoreRead  DataStoreName=MotAg0PrevRollgCntr
  RollgCntr : Outport
  wires:
  Data Store Read/1 -> RollgCntr/1

== system CM620C_MotAg0Meas/MotAg0Meas/MotAg0MeasPer2/MotAg0Calcn/MotAg0Processing/Diagnostics/Rolling Counter/Test Pass ==
  Action Port : ActionPort  ActionType=then
  CopyRight2 : Subsystem  Description=|  mask(Copyright Information){none=on}
      | Copyright info block.                                               
      |                                                                     
      | Place copyright information at the top of every subsystem in design.
      mask prompts: none "No parameters"
      mask help: Place copyright information at the top of every subsystem in design.
      mask Display:
      | NxtrConf = 'Nexteer Confidential';
      | 
      | sys = bdroot; %handle for the current model ("system")
      | first = get_param(sys,'Created');
      | first = first(end-3:end);  %year is last four digits
      | 
      | last = get_param(sys,'LastModifiedDate');
      | if isempty(last)
      |     last = datestr(now,'yyyy');
      | else
      |     last = last(end-3:end);
      | end
      | 
      | if strcmp(first,last)
      |     fprintf('%s -- Copyright %s Nexteer',NxtrConf,first)
      | else
      |     fprintf('%s -- %s%s- %s Nexteer',NxtrConf,char(169),first,last)
      | end
  Data Store Read : DataStoreRead  DataStoreName=MotAg0PrevRollgCntr
  If : If  IfExpression=u1==255
  Merge : Merge
  Wrap back to 0 : Subsystem  TreatAsAtomicUnit=on
  i++ : Subsystem  TreatAsAtomicUnit=on
  RollgCntr : Outport
  wires:
  Data Store Read/1 -> If/1
  If/1 -> Wrap back to 0/Action
  If/2 -> i++/Action
  Wrap back to 0/1(RollgCntr) -> Merge/1
  i++/1(RollgCntr) -> Merge/2
  Merge/1 -> RollgCntr/1

== system CM620C_MotAg0Meas/MotAg0Meas/MotAg0MeasPer2/MotAg0Calcn/MotAg0Processing/Diagnostics/SPI vs ENCA/CopyRight2 ==

== system CM620C_MotAg0Meas/MotAg0Meas/MotAg0MeasPer2/MotAg0Calcn/MotAg0Processing/Diagnostics/SPI vs ENCA/No Error ==
  Action Port : ActionPort  ActionType=else
  Constant : Constant  Value=0  OutDataTypeStr=boolean
  CopyRight2 : Subsystem  Description=|  mask(Copyright Information){none=on}
      | Copyright info block.                                               
      |                                                                     
      | Place copyright information at the top of every subsystem in design.
      mask prompts: none "No parameters"
      mask help: Place copyright information at the top of every subsystem in design.
      mask Display:
      | NxtrConf = 'Nexteer Confidential';
      | 
      | sys = bdroot; %handle for the current model ("system")
      | first = get_param(sys,'Created');
      | first = first(end-3:end);  %year is last four digits
      | 
      | last = get_param(sys,'LastModifiedDate');
      | if isempty(last)
      |     last = datestr(now,'yyyy');
      | else
      |     last = last(end-3:end);
      | end
      | 
      | if strcmp(first,last)
      |     fprintf('%s -- Copyright %s Nexteer',NxtrConf,first)
      | else
      |     fprintf('%s -- %s%s- %s Nexteer',NxtrConf,char(169),first,last)
      | end
  AgErr : Outport
  wires:
  Constant/1 -> AgErr/1

== system CM620C_MotAg0Meas/MotAg0Meas/MotAg0MeasPer2/MotAg0Calcn/MotAg0Processing/Diagnostics/SPI vs ENCA/Sub 0 ==
  Inp : Inport
  Action Port : ActionPort  ActionType=else
  CopyRight2 : Subsystem  Description=|  mask(Copyright Information){none=on}
      | Copyright info block.                                               
      |                                                                     
      | Place copyright information at the top of every subsystem in design.
      mask prompts: none "No parameters"
      mask help: Place copyright information at the top of every subsystem in design.
      mask Display:
      | NxtrConf = 'Nexteer Confidential';
      | 
      | sys = bdroot; %handle for the current model ("system")
      | first = get_param(sys,'Created');
      | first = first(end-3:end);  %year is last four digits
      | 
      | last = get_param(sys,'LastModifiedDate');
      | if isempty(last)
      |     last = datestr(now,'yyyy');
      | else
      |     last = last(end-3:end);
      | end
      | 
      | if strcmp(first,last)
      |     fprintf('%s -- Copyright %s Nexteer',NxtrConf,first)
      | else
      |     fprintf('%s -- %s%s- %s Nexteer',NxtrConf,char(169),first,last)
      | end
  Outp : Outport
  wires:
  Inp/1 -> Outp/1

== system CM620C_MotAg0Meas/MotAg0Meas/MotAg0MeasPer2/MotAg0Calcn/MotAg0Processing/Diagnostics/SPI vs ENCA/Sub 65535 ==
  Inp : Inport
  Action Port : ActionPort  ActionType=then
  CopyRight2 : Subsystem  Description=|  mask(Copyright Information){none=on}
      | Copyright info block.                                               
      |                                                                     
      | Place copyright information at the top of every subsystem in design.
      mask prompts: none "No parameters"
      mask help: Place copyright information at the top of every subsystem in design.
      mask Display:
      | NxtrConf = 'Nexteer Confidential';
      | 
      | sys = bdroot; %handle for the current model ("system")
      | first = get_param(sys,'Created');
      | first = first(end-3:end);  %year is last four digits
      | 
      | last = get_param(sys,'LastModifiedDate');
      | if isempty(last)
      |     last = datestr(now,'yyyy');
      | else
      |     last = last(end-3:end);
      | end
      | 
      | if strcmp(first,last)
      |     fprintf('%s -- Copyright %s Nexteer',NxtrConf,first)
      | else
      |     fprintf('%s -- %s%s- %s Nexteer',NxtrConf,char(169),first,last)
      | end
  Outp : Outport
  wires:
  Inp/1 -> Outp/1

== system CM620C_MotAg0Meas/MotAg0Meas/MotAg0MeasPer2/MotAg0Calcn/MotAg0Processing/Diagnostics/SPI vs ENCA/Sync Error ==
  Action Port : ActionPort  ActionType=then
  Constant : Constant  OutDataTypeStr=boolean
  CopyRight2 : Subsystem  Description=|  mask(Copyright Information){none=on}
      | Copyright info block.                                               
      |                                                                     
      | Place copyright information at the top of every subsystem in design.
      mask prompts: none "No parameters"
      mask help: Place copyright information at the top of every subsystem in design.
      mask Display:
      | NxtrConf = 'Nexteer Confidential';
      | 
      | sys = bdroot; %handle for the current model ("system")
      | first = get_param(sys,'Created');
      | first = first(end-3:end);  %year is last four digits
      | 
      | last = get_param(sys,'LastModifiedDate');
      | if isempty(last)
      |     last = datestr(now,'yyyy');
      | else
      |     last = last(end-3:end);
      | end
      | 
      | if strcmp(first,last)
      |     fprintf('%s -- Copyright %s Nexteer',NxtrConf,first)
      | else
      |     fprintf('%s -- %s%s- %s Nexteer',NxtrConf,char(169),first,last)
      | end
  AgErr : Outport
  wires:
  Constant/1 -> AgErr/1

== system CM620C_MotAg0Meas/MotAg0Meas/MotAg0MeasPer2/MotAg0Calcn/MotAg0Processing/Diagnostics/SetParamByte/Boolean to u8 ==
  InputBoolean : Inport  OutDataTypeStr=boolean
  CopyRight2 : Subsystem  Description=|  mask(Copyright Information){none=on}
      | Copyright info block.                                               
      |                                                                     
      | Place copyright information at the top of every subsystem in design.
      mask prompts: none "No parameters"
      mask help: Place copyright information at the top of every subsystem in design.
      mask Display:
      | NxtrConf = 'Nexteer Confidential';
      | 
      | sys = bdroot; %handle for the current model ("system")
      | first = get_param(sys,'Created');
      | first = first(end-3:end);  %year is last four digits
      | 
      | last = get_param(sys,'LastModifiedDate');
      | if isempty(last)
      |     last = datestr(now,'yyyy');
      | else
      |     last = last(end-3:end);
      | end
      | 
      | if strcmp(first,last)
      |     fprintf('%s -- Copyright %s Nexteer',NxtrConf,first)
      | else
      |     fprintf('%s -- %s%s- %s Nexteer',NxtrConf,char(169),first,last)
      | end
  If : If  IfExpression=u1 ~= 0
  Merge : Merge
  Output 0 : Subsystem  TreatAsAtomicUnit=on
  Output 1 : Subsystem  TreatAsAtomicUnit=on
  OutputNumber : Outport  OutDataTypeStr=uint8
  wires:
  InputBoolean/1 -> If/1
  If/1 -> Output 1/Action
  If/2 -> Output 0/Action
  Output 1/1(Out1) -> Merge/1
  Output 0/1(Out1) -> Merge/2
  Merge/1 -> OutputNumber/1

== system CM620C_MotAg0Meas/MotAg0Meas/MotAg0MeasPer2/MotAg0Calcn/MotAg0Processing/Diagnostics/SetParamByte/Boolean to u8  ==
  InputBoolean : Inport  OutDataTypeStr=boolean
  CopyRight2 : Subsystem  Description=|  mask(Copyright Information){none=on}
      | Copyright info block.                                               
      |                                                                     
      | Place copyright information at the top of every subsystem in design.
      mask prompts: none "No parameters"
      mask help: Place copyright information at the top of every subsystem in design.
      mask Display:
      | NxtrConf = 'Nexteer Confidential';
      | 
      | sys = bdroot; %handle for the current model ("system")
      | first = get_param(sys,'Created');
      | first = first(end-3:end);  %year is last four digits
      | 
      | last = get_param(sys,'LastModifiedDate');
      | if isempty(last)
      |     last = datestr(now,'yyyy');
      | else
      |     last = last(end-3:end);
      | end
      | 
      | if strcmp(first,last)
      |     fprintf('%s -- Copyright %s Nexteer',NxtrConf,first)
      | else
      |     fprintf('%s -- %s%s- %s Nexteer',NxtrConf,char(169),first,last)
      | end
  If : If  IfExpression=u1 ~= 0
  Merge : Merge
  Output 0 : Subsystem  TreatAsAtomicUnit=on
  Output 1 : Subsystem  TreatAsAtomicUnit=on
  OutputNumber : Outport  OutDataTypeStr=uint8
  wires:
  Merge/1 -> OutputNumber/1
  Output 0/1(Out1) -> Merge/2
  Output 1/1(Out1) -> Merge/1
  If/2 -> Output 0/Action
  If/1 -> Output 1/Action
  InputBoolean/1 -> If/1
